simulink model "hw3_sim"  (R2018b)
settings: Solver=VariableStepAuto  StartTime=0.0  StopTime=10.0  RelTol=1e-3
values from neighbouring files (symbols this model uses):
  B = 0    [hw4.m]    (also in hw4_main.m; hw4_q1.m; hw4_q2.m = 0.1; hw4_q3.m)
  g = 9.8    [hw4.m]    (also in hw4_main.m; hw4_q1.m; hw4_q2.m; hw4_q3.m)
  K1 = 20    [hw4.m]    (also in hw4_main.m; hw4_q1.m; hw4_q2.m; hw4_q3.m)
  L = L1 + L2    (= 0.5)    [hw4.m]    (also in hw4_main.m; hw4_q1.m; hw4_q2.m; hw4_q3.m)
  L1 = 0.25    [hw4.m]    (also in hw4_main.m; hw4_q1.m; hw4_q2.m; hw4_q3.m)
  M1 = 10    [hw4.m]    (also in hw4_main.m; hw4_q1.m; hw4_q2.m; hw4_q3.m)
  M2 = 10    [hw4.m]    (also in hw4_main.m; hw4_q1.m; hw4_q2.m; hw4_q3.m)
settings Model: Creator=CHENG  LastModifiedBy=CHENG

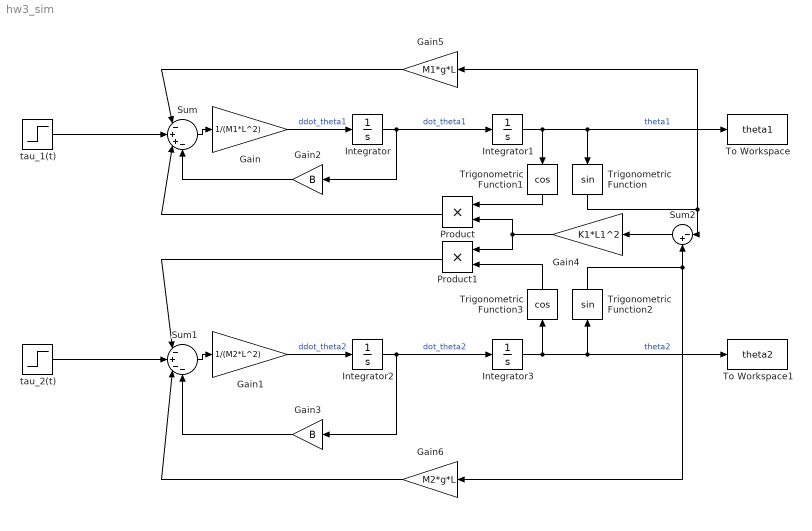
== system hw3_sim ==
  Gain : Gain  Gain=1/(M1*L^2)
  Gain1 : Gain  Gain=1/(M2*L^2)
  Gain2 : Gain  Gain=B
  Gain3 : Gain  Gain=B
  Gain4 : Gain  Gain=K1*L1^2
  Gain5 : Gain  Gain=M1*g*L
  Gain6 : Gain  Gain=M2*g*L
  Integrator{,1..3} (4 alike) : Integrator
  Product : Product
  Product1 : Product
  Sum : Sum  Inputs=|-++-
  Sum1 : Sum  Inputs=|-+--
  Sum2 : Sum  Inputs=|-+
  To Workspace : ToWorkspace  VariableName=theta1  SaveFormat=Timeseries  SampleTime=-1
  To Workspace1 : ToWorkspace  VariableName=theta2  SaveFormat=Timeseries  SampleTime=-1
  Trigonometric Function : Trigonometry
  Trigonometric Function1 : Trigonometry  Operator=cos
  Trigonometric Function2 : Trigonometry
  Trigonometric Function3 : Trigonometry  Operator=cos
  tau_1(t) : Step  SampleTime=0
  tau_2(t) : Step  SampleTime=0
  wires:
  Integrator/1 -> Gain2/1, Integrator1/1  "dot_theta1"
  Gain/1 -> Integrator/1  "ddot_theta1"
  Sum/1 -> Gain/1
  Integrator1/1 -> Trigonometric Function1/1, Trigonometric Function/1, To Workspace/1  "theta1"
  Integrator3/1 -> Trigonometric Function3/1, Trigonometric Function2/1, To Workspace1/1  "theta2"
  Sum1/1 -> Gain1/1
  tau_2(t)/1 -> Sum1/2
  Gain1/1 -> Integrator2/1  "ddot_theta2"
  Integrator2/1 -> Gain3/1, Integrator3/1  "dot_theta2"
  Gain2/1 -> Sum/4
  Gain3/1 -> Sum1/4
  Trigonometric Function/1 -> Gain5/1, Sum2/1
  Sum2/1 -> Gain4/1
  Trigonometric Function3/1 -> Product1/2
  Trigonometric Function1/1 -> Product/1
  Gain4/1 -> Product/2, Product1/1
  Product/1 -> Sum/3
  tau_1(t)/1 -> Sum/2
  Gain5/1 -> Sum/1
  Trigonometric Function2/1 -> Gain6/1, Sum2/2
  Gain6/1 -> Sum1/3
  Product1/1 -> Sum1/1
